simulink model "lab2sim"  (Simulink 10.2)
settings: Solver=ode45  StartTime=0.0  StopTime=30  RelTol=1e-3  EnableMultiTasking=on
libraries: ELE819m x1
settings Model: Creator=Admin  LastModifiedBy=djclarke
settings DataIOCC: LimitDataPoints=on
settings OptimizationCC: ExpressionDepthLimit=2147483647
settings DebuggingCC: AlgebraicLoopMsg=none  ArtificialAlgebraicLoopMsg=none  StateNameClashWarn=warning
settings SFSimCC: SimParseCustomCode=off

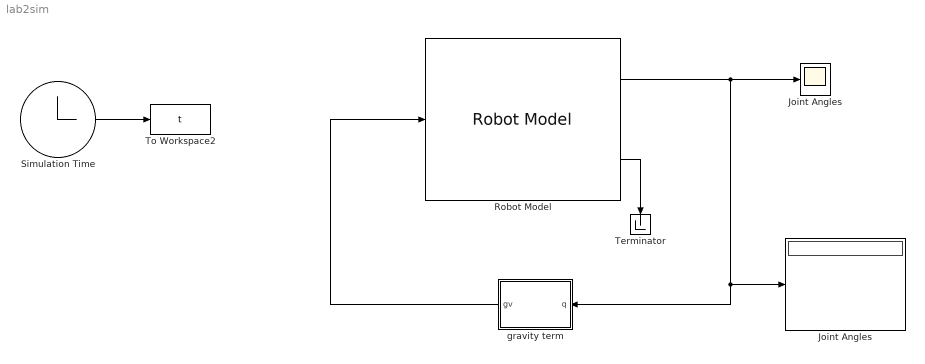
== system lab2sim ==
  Joint Angles : Scope
  "Joint Angles " : Display
  Robot Model : ELE819m/Robot Model  q1_0=pi/9  q2_0=pi/3  q3_0=-pi/2
  Simulation Time : Clock
      settings: Decimation=200
  Terminator : Terminator
  To Workspace2 : ToWorkspace  VariableName=t  SampleTime=-1
      settings: Decimation=200
  gravity term : MATLAB Function  TreatAsAtomicUnit=on
  wires:
  Robot Model/1 -> "Joint Angles "/1, gravity term/1(q), Joint Angles/1
  Simulation Time/1 -> To Workspace2/1
  gravity term/1(gv) -> Robot Model/1
  Robot Model/2 -> Terminator/1

== matlab function gravity term ==
  data: q input double; gv output double
function gv = grav_em(q)
    q2 = q(2); q3 = q(3);
    
    g = 9.81;
    
    m2 = 0.035; m3 = 0.1;
    l2 = 0.13335; l3 = 0.13335;
    lc2 = 0.5*l2; lc3 = 0.9*l3;
   
    g1 = 0;
    g2 = m2*g*lc2*cos(q2) + m3*g*l2*cos(q2) + m3*g*lc3*cos(q2 + q3);
    g3 = m3*g*lc3*cos(q2 + q3);
    
    gv = [g1 g2 g3];
end
